simulink model "Environment_Full"  (R2016b)
settings: Solver=VariableStepAuto  StartTime=0.0  StopTime=10.0  RelTol=1e-3
values from neighbouring files (symbols this model uses):
  Env =     [UAV_modelconfig.mat]
libraries: Environment_Lib x2, aerolibatmos2 x1, aerolibgravity2 x1
settings Model: Creator=UAVLAB  LastModifiedBy=UAVLAB

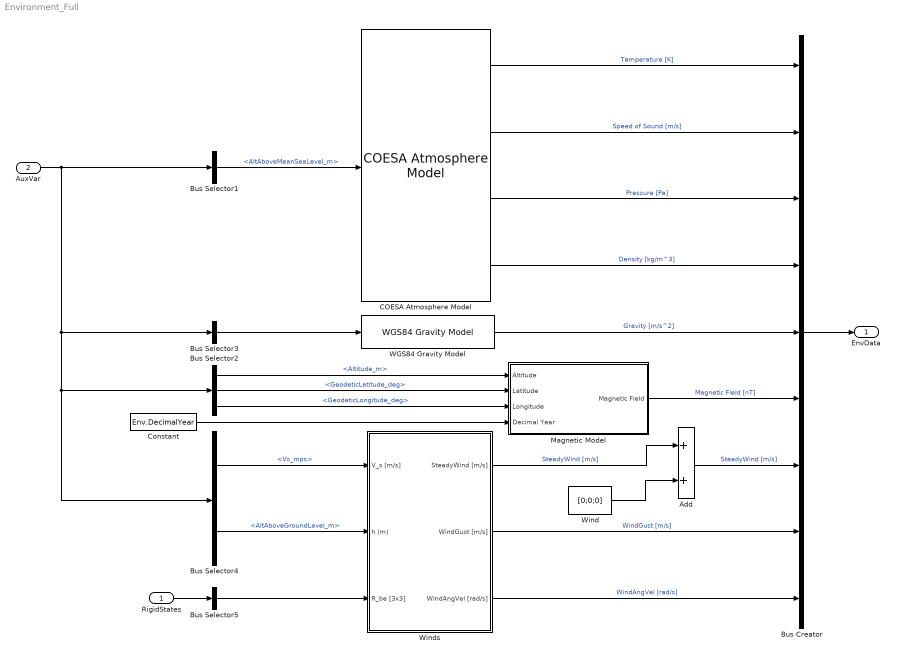
== system Environment_Full ==
  RigidStates : Inport  OutDataTypeStr=Bus: RigidStates
  AuxVar : Inport  Port=2  OutDataTypeStr=Bus: AuxVar
  Add : Sum
  Bus Creator : BusCreator  Inputs=9  OutDataTypeStr=Bus: EnvData
      settings: InheritFromInputs=off
  Bus Selector1 : BusSelector  OutputSignals=Nav.AltAboveMeanSeaLevel_m
  Bus Selector2 : BusSelector  OutputSignals=Nav.Altitude_m,Nav.GeodeticLatitude_deg,Nav.GeodeticLongitude_deg
  Bus Selector3 : BusSelector  OutputSignals=Nav.GeodeticLatitude_deg,Nav.GeodeticLongitude_deg,Nav.Altitude_m  OutputAsBus=on
  Bus Selector4 : BusSelector  OutputSignals=WindAxesParams.Vs_mps,Nav.AltAboveGroundLevel_m
  Bus Selector5 : BusSelector  OutputSignals=DCM  OutputAsBus=on
  COESA Atmosphere Model : aerolibatmos2/COESA Atmosphere Model  units=Metric (MKS)  spec=1976 COESA-extended U.S. Standard Atmosphere  model=Profile  profile_var=High temperature  profile_percent=1%  profile_alt=5 km (16404 ft)  envelope_var=High temperature  envelope_percent=1%  action=Warning
  Constant : Constant  Value=Env.DecimalYear
  Magnetic Model : Subsystem  BlockChoice=WMM Bypass
      settings: AttributesFormatString=%<BlockChoice>  TemplateBlock=Environment_Lib/Magnetic Model  MemberBlocks=WMM 2005,WMM Bypass
  "WGS84 Gravity Model " : aerolibgravity2/WGS84 Gravity Model   model=WGS84 Taylor Series  units=Metric (MKS)  no_atmos=on  precessing=on  jd_loc=off  month=October  day=10  year=2004  no_centrifugal=on  action=Warning
  Wind : Constant  Value=[0;0;0]
  Winds : Subsystem  BlockChoice=Wind Bypass
      settings: AttributesFormatString=%<BlockChoice>  TemplateBlock=Environment_Lib/Winds  MemberBlocks=Wind & Turbulence,Wind Bypass
  EnvData : Outport  OutDataTypeStr=Bus: EnvData
  wires:
  Winds/1(SteadyWind [m/s]) -> Add/1  "SteadyWind [m/s]"
  Wind/1 -> Add/2
  Winds/3(WindAngVel [rad/s]) -> Bus Creator/9  "WindAngVel [rad/s]"
  Winds/2(WindGust [m/s]) -> Bus Creator/8  "WindGust [m/s]"
  Add/1 -> Bus Creator/7  "SteadyWind [m/s]"
  Magnetic Model/1(Magnetic Field) -> Bus Creator/6  "Magnetic Field [nT]"
  "WGS84 Gravity Model "/1 -> Bus Creator/5  "Gravity [m/s^2]"
  Bus Selector5/1 -> Winds/3(R_be [3x3])
  RigidStates/1 -> Bus Selector5/1
  AuxVar/1 -> Bus Selector1/1, Bus Selector2/1, Bus Selector4/1, Bus Selector3/1
  Constant/1 -> Magnetic Model/4(Decimal Year)
  Bus Selector3/1 -> "WGS84 Gravity Model "/1
  Bus Selector2/3 -> Magnetic Model/3(Longitude)  "<GeodeticLongitude_deg>"
  Bus Selector2/2 -> Magnetic Model/2(Latitude)  "<GeodeticLatitude_deg>"
  Bus Selector2/1 -> Magnetic Model/1(Altitude)  "<Altitude_m>"
  COESA Atmosphere Model/4 -> Bus Creator/4  "Density [kg/m^3]"
  COESA Atmosphere Model/1 -> Bus Creator/1  "Temperature [K]"
  COESA Atmosphere Model/2 -> Bus Creator/2  "Speed of Sound [m/s]"
  COESA Atmosphere Model/3 -> Bus Creator/3  "Pressure [Pa]"
  Bus Selector1/1 -> COESA Atmosphere Model/1  "<AltAboveMeanSeaLevel_m>"
  Bus Creator/1 -> EnvData/1
  Bus Selector4/1 -> Winds/1(V_s [m/s])  "<Vs_mps>"
  Bus Selector4/2 -> Winds/2(h (m))  "<AltAboveGroundLevel_m>"

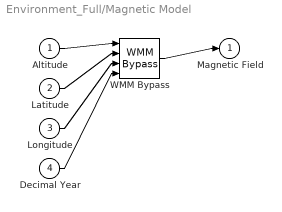
== system Environment_Full/Magnetic Model ==
  Altitude : Inport
  Latitude : Inport  Port=2
  Longitude : Inport  Port=3
  Decimal Year : Inport  Port=4
  WMM Bypass : Environment_Lib/WMM Bypass  units=Metric (MKS)  time_in=on  month=August  day=1  year=2009  action=None  h_out=off  dec_out=off  inc_out=off  ti_out=off
  Magnetic Field : Outport
  wires:
  Altitude/1 -> WMM Bypass/1
  Latitude/1 -> WMM Bypass/2
  Longitude/1 -> WMM Bypass/3
  Decimal Year/1 -> WMM Bypass/4
  WMM Bypass/1 -> Magnetic Field/1

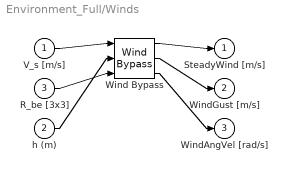
== system Environment_Full/Winds ==
  V_s [m/s] : Inport
  h (m) : Inport  Port=2
  R_be [3x3] : Inport  Port=3
  Wind Bypass : Environment_Lib/Wind Bypass
  SteadyWind [m/s] : Outport
  WindGust [m/s] : Outport  Port=2
  WindAngVel [rad/s] : Outport  Port=3
  wires:
  V_s [m/s]/1 -> Wind Bypass/1
  h (m)/1 -> Wind Bypass/2
  R_be [3x3]/1 -> Wind Bypass/3
  Wind Bypass/1 -> SteadyWind [m/s]/1
  Wind Bypass/2 -> WindGust [m/s]/1
  Wind Bypass/3 -> WindAngVel [rad/s]/1
